simulink model "balance_car_with_NN"  (R2023b)
settings: Solver=VariableStepAuto  StartTime=0.0  StopTime=100  RelTol=1e-3
values from neighbouring files (symbols this model uses):
  d = 0.1612    [new_parameter.m]    (also in parameter.m)
  g = 9.8    [new_parameter.m]    (also in parameter.m)
  I = 0.5*m*r^2    (= 1.3475e-05)    [new_parameter.m]    (also in parameter.m = 1.97568e-05)
  J_delta = (1/12)*M*(0.0930^2+0.0530^2)    (= 0.000680796166667)    [new_parameter.m]    (also in parameter.m = 0.0006559705)
  J_p = (1/12)*M*(0.3^2+0.08^2)    (= 0.00572776666667)    [new_parameter.m]    (also in parameter.m = 0.0006276369025)
  l = 0.5*0.8    (= 0.4)    [new_parameter.m]    (also in parameter.m = 0.04515)
  M = 0.757-2*m    (= 0.713)    [new_parameter.m]    (also in parameter.m = 0.687)
  m = 0.022    [new_parameter.m]    (also in parameter.m = 0.035)
  r = 0.07/2    (= 0.035)    [new_parameter.m]    (also in parameter.m = 0.0336)
  T = evalin('base', 'T')    [NN_controller.m]    (also in new_parameter.m = 0.01; parameter.m = 0.02)
undefined symbols (not defined in the file or in its folder): now
libraries: slpidlib x7, simulink x6, cstblocks x1
settings Model: Creator=zhy  LastModifiedBy=zhy

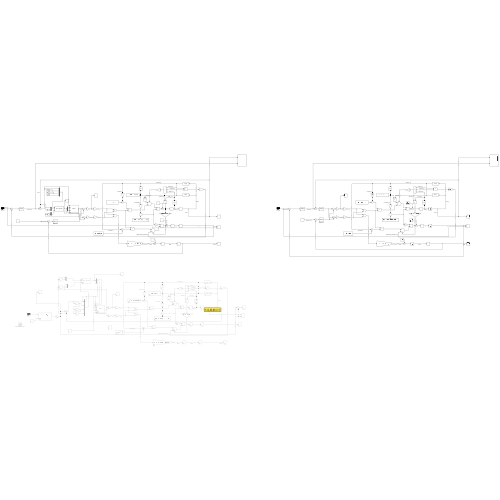
[thumbnail: Simulink's stored preview of the top-level diagram]
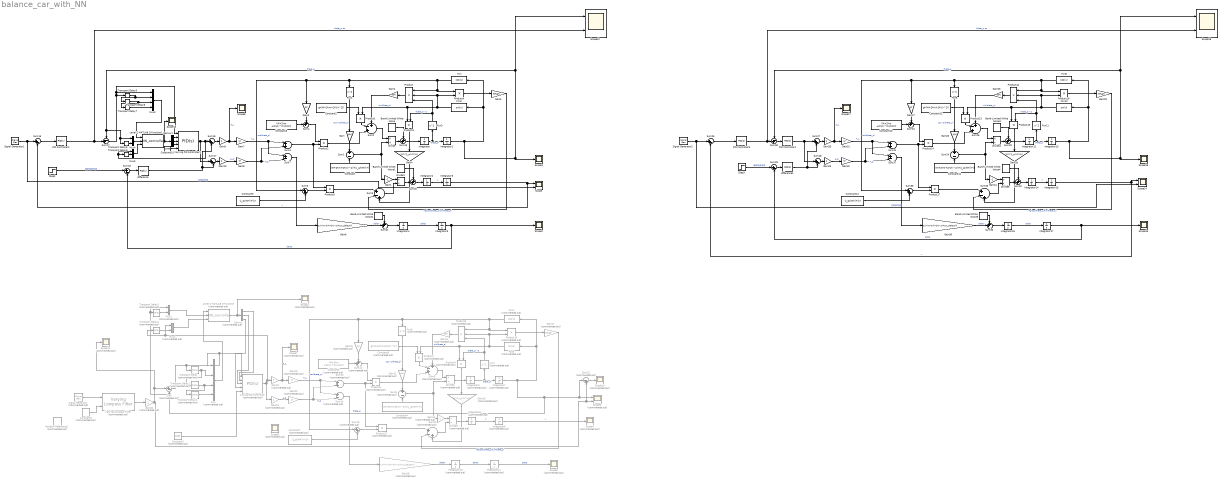
== system balance_car_with_NN ==
  Band-Limited White Noise : simulink/Sources/Band-Limited White Noise  Cov=[0.00001]  Ts=0.1  seed=[23341]
  Band-Limited White Noise1 : simulink/Sources/Band-Limited White Noise  Cov=[0.00001]  Ts=0.1  seed=[23342]
  Band-Limited White Noise2 : simulink/Sources/Band-Limited White Noise  Cov=[0.0001]  Ts=0.1  seed=[23343]
  Band-Limited White Noise3 : simulink/Sources/Band-Limited White Noise  Cov=[0.00001]  Ts=0.1  seed=[23341]
  Band-Limited White Noise4 : simulink/Sources/Band-Limited White Noise  Cov=[0.00001]  Ts=0.1  seed=[23342]
  Band-Limited White Noise5 : simulink/Sources/Band-Limited White Noise  Cov=[0.0001]  Ts=0.1  seed=[23343]
  Constant : Constant  Value=(M+2*m+2*I/(r^2))*(J_p/(M*l)+l)
  Constant1 : Constant  Commented=on  Value=1000
  Constant10 : Constant  Value=1000
  Constant11 : Constant  Value=(M+2*m+2*I/(r^2))*(J_p/(M*l)+l)
  Constant12 : Constant  Value=g*(M+2*m+2*I/(r^2))
  Constant13 : Constant  Value=(M+2*m +2*I/(r^2))/(M*l)
  Constant14 : Constant  Value=(J_p/(M*l)+l)/r
  Constant2 : Constant  Value=g*(M+2*m+2*I/(r^2))
  Constant3 : Constant  Value=(M+2*m +2*I/(r^2))/(M*l)
  Constant4 : Constant  Commented=on  Value=(M+2*m+2*I/(r^2))*(J_p/(M*l)+l)
  Constant5 : Constant  Commented=on  Value=g*(M+2*m+2*I/(r^2))
  Constant6 : Constant  Commented=on  Value=(M+2*m +2*I/(r^2))/(M*l)
  Constant7 : Constant  Commented=on  Value=(J_p/(M*l)+l)/r
  Constant8 : Constant  Commented=on  Value=0.05*pi
  Constant9 : Constant  Value=(J_p/(M*l)+l)/r
  Demux : Demux  Commented=on  Outputs=3
  Demux1 : Demux  Outputs=3
  Divide : Product  Inputs=*/
  Divide1 : Product  Inputs=/*
  Divide2 : Product  Commented=on  Inputs=*/
  Divide3 : Product  Commented=on  Inputs=/*
  Divide4 : Product  Inputs=*/
  Divide5 : Product  Inputs=/*
  Fcn : Fcn  Expr=cos(u)
  Fcn{1,3,9,11} (4 alike) : Fcn  Expr=u^2
  Fcn10 : Fcn  Expr=sin(u)
  Fcn2 : Fcn  Expr=sin(u)
  Fcn4 : Fcn  Commented=on  Expr=cos(u)
  Fcn5 : Fcn  Commented=on  Expr=u^2
  Fcn6 : Fcn  Commented=on  Expr=sin(u)
  Fcn7 : Fcn  Commented=on  Expr=u^2
  Fcn8 : Fcn  Expr=cos(u)
  Gain{,2,23,26} (4 alike) : Gain  Gain=M*l
  Gain1 : Gain  Gain=-1
  Gain{9..10,25,33} (4 alike) : Gain
  Gain11 : Gain  Commented=on  Gain=M*l
  Gain12 : Gain  Commented=on  Gain=-1
  Gain13 : Gain  Commented=on
  Gain14 : Gain  Commented=on  Gain=M*l
  Gain15 : Gain  Commented=on  Gain=1/r
  Gain16 : Gain  Commented=on  Gain=(M*l)*(J_p/(M*l)+l)
  Gain17 : Gain  Commented=on  Gain=M*g*l
  Gain18 : Gain  Commented=on  Gain=1/(r*(m*d+I*d/(r^2)+2*J_delta/d))
  Gain19 : Gain  Commented=on  Gain=I/r
  Gain20 : Gain  Commented=on  Gain=I/r
  Gain21 : Gain  Commented=on
  Gain22 : Gain  Commented=on
  Gain24 : Gain  Gain=-1
  Gain27 : Gain  Gain=1/r
  Gain28 : Gain  Gain=(M*l)*(J_p/(M*l)+l)
  Gain29 : Gain  Gain=M*g*l
  Gain3 : Gain  Gain=1/r
  Gain30 : Gain  Gain=1/(r*(m*d+I*d/(r^2)+2*J_delta/d))
  Gain{7..8,31..32} (4 alike) : Gain  Gain=I/r
  Gain4 : Gain  Gain=(M*l)*(J_p/(M*l)+l)
  Gain5 : Gain  Gain=M*g*l
  Gain6 : Gain  Gain=1/(r*(m*d+I*d/(r^2)+2*J_delta/d))
  Integrator{,1..5,12..17} (12 alike) : Integrator
  Integrator{6..11} (6 alike) : Integrator  Commented=on
  Level-2 MATLAB S-Function : M-S-Function  Commented=on  FunctionName=NN_controller
  Level-2 MATLAB S-Function1 : M-S-Function  FunctionName=NN_controller
  Mux : Mux  Commented=on
  Mux1 : Mux  Commented=on  Inputs=2
  Mux2 : Mux  Commented=on  Inputs=2
  Mux3 : Mux
  Mux4 : Mux  Inputs=2
  Mux5 : Mux  Inputs=2
  PID Controller1 : slpidlib/PID Controller  Controller=PID  Form=Parallel  TimeDomain=Continuous-time  UseExternalTs=off  SampleTime=-1  IntegratorMethod=Forward Euler  FilterMethod=Forward Euler  ControllerParametersSource=internal  P=-280  I=-200  UseKiTs=off  D=-120  N=100000  UseFilter=on  TunerSelectOption=Transfer Function Based (PID Tuner App)  InitialConditionSource=internal  InitialConditionForIntegrator=0  InitialConditionForFilter=0  DifferentiatorICPrevScaledInput=0  ExternalReset=none  TrackingMode=off  Kt=1  LimitOutput=off  SatLimitsSource=internal  UpperSaturationLimit=inf  LowerSaturationLimit=-inf  LinearizeAsGain=on  AntiWindupMode=none  Kb=1  LimitIntegrator=off  UpperIntegratorSaturationLimit=inf  LowerIntegratorSaturationLimit=-inf  POutMin=[]  POutMax=[]  IOutMin=[]  IOutMax=[]  DOutMin=[]  DOutMax=[]  NOutMin=[]  NOutMax=[]  SumOutMin=[]  SumOutMax=[]  SaturationOutMin=[]  SaturationOutMax=[]  PParamMin=[]  PParamMax=[]  IParamMin=[]  IParamMax=[]  DParamMin=[]  DParamMax=[]  NParamMin=[]  NParamMax=[]  KbParamMin=[]  KbParamMax=[]  KtParamMin=[]  KtParamMax=[]  KbOutMin=[]  KbOutMax=[]  KtOutMin=[]  KtOutMax=[]  IntegratorOutMin=[]  IntegratorOutMax=[]  FilterOutMin=[]  FilterOutMax=[]  SumI1OutMin=[]  SumI1OutMax=[]  SumI2OutMin=[]  SumI2OutMax=[]  SumI3OutMin=[]  SumI3OutMax=[]  SumI4OutMin=[]  SumI4OutMax=[]  SumDOutMin=[]  SumDOutMax=[]  DifferentiatorOutMin=[]  DifferentiatorOutMax=[]  FilterDiffOutCoefMin=[]  FilterDiffOutCoefMax=[]  ReciprocalOutMin=[]  ReciprocalOutMax=[]  SumDenOutMin=[]  SumDenOutMax=[]  SumNumOutMin=[]  SumNumOutMax=[]  DivideOutMin=[]  DivideOutMax=[]  UdiffTsProdOutMin=[]  UdiffTsProdOutMax=[]  NTsProdOutMin=[]  NTsProdOutMax=[]  UintegralTsProdOutMin=[]  UintegralTsProdOutMax=[]  UngainTsProdOutMin=[]  UngainTsProdOutMax=[]  ClampingZeroOutDataTypeStr=Inherit: Inherit via back propagation  ClampingZeroOutMin=[]  ClampingZeroOutMax=[]  FilterDenConstantOutDataTypeStr=Inherit: Inherit via back propagation  FilterDenConstantOutMin=[]  FilterDenConstantOutMax=[]  PCopyOutDataTypeStr=Inherit: Inherit via back propagation  PCopyOutMin=[]  PCopyOutMax=[]  NCopyOutDataTypeStr=Inherit: Inherit via back propagation  NCopyOutMin=[]  NCopyOutMax=[]  IntegratorContinuousStateAttributes=''  IntegratorStateMustResolveToSignalObject=off  IntegratorRTWStateStorageClass=Auto  FilterContinuousStateAttributes=''  FilterStateMustResolveToSignalObject=off  FilterRTWStateStorageClass=Auto  ParallelPVariant=InternalParameters  IdealPVariant=Disabled  IVariant=InternalParameters  DVariant=InternalParameters  IntegratorVariant=Continuous  SatVariant=Disabled  AWVariant=Passthrough  PCopyVariant=Disabled  TRVariant=Disabled  FdbkBlocksVariant=Forward  IdealPFdbkVariant=Disabled  SatFdbkVariant=Disabled  DerivativeFilterVariant=ContFilter  NVariant=InternalParameters  NCopyVariant=Disabled  FilterICVariant=InternalICsFilter  IntegratorICVariant=InternalICs  ExternalResetVariant=Disabled  TRSumVariant=Passthrough  SumFdbkVariant=Disabled  SumVariant=Sum_PID  TsampFilterVariant=InternalTs  TsampNgainVariant=Passthrough  TsampIntegralVariant=Disabled_SignalSpec  ExternalSaturationOutDataTypeStr=Inherit: Same as second input
  PID Controller2 : slpidlib/PID Controller  Controller=PID  Form=Parallel  TimeDomain=Continuous-time  UseExternalTs=off  SampleTime=-1  IntegratorMethod=Forward Euler  FilterMethod=Forward Euler  ControllerParametersSource=internal  P=0.01  I=0  UseKiTs=off  D=0.2  N=1  UseFilter=on  TunerSelectOption=Transfer Function Based (PID Tuner App)  InitialConditionSource=internal  InitialConditionForIntegrator=0  InitialConditionForFilter=0  DifferentiatorICPrevScaledInput=0  ExternalReset=none  TrackingMode=off  Kt=1  LimitOutput=off  SatLimitsSource=internal  UpperSaturationLimit=inf  LowerSaturationLimit=-inf  LinearizeAsGain=on  AntiWindupMode=none  Kb=1  LimitIntegrator=off  UpperIntegratorSaturationLimit=inf  LowerIntegratorSaturationLimit=-inf  POutMin=[]  POutMax=[]  IOutMin=[]  IOutMax=[]  DOutMin=[]  DOutMax=[]  NOutMin=[]  NOutMax=[]  SumOutMin=[]  SumOutMax=[]  SaturationOutMin=[]  SaturationOutMax=[]  PParamMin=[]  PParamMax=[]  IParamMin=[]  IParamMax=[]  DParamMin=[]  DParamMax=[]  NParamMin=[]  NParamMax=[]  KbParamMin=[]  KbParamMax=[]  KtParamMin=[]  KtParamMax=[]  KbOutMin=[]  KbOutMax=[]  KtOutMin=[]  KtOutMax=[]  IntegratorOutMin=[]  IntegratorOutMax=[]  FilterOutMin=[]  FilterOutMax=[]  SumI1OutMin=[]  SumI1OutMax=[]  SumI2OutMin=[]  SumI2OutMax=[]  SumI3OutMin=[]  SumI3OutMax=[]  SumI4OutMin=[]  SumI4OutMax=[]  SumDOutMin=[]  SumDOutMax=[]  DifferentiatorOutMin=[]  DifferentiatorOutMax=[]  FilterDiffOutCoefMin=[]  FilterDiffOutCoefMax=[]  ReciprocalOutMin=[]  ReciprocalOutMax=[]  SumDenOutMin=[]  SumDenOutMax=[]  SumNumOutMin=[]  SumNumOutMax=[]  DivideOutMin=[]  DivideOutMax=[]  UdiffTsProdOutMin=[]  UdiffTsProdOutMax=[]  NTsProdOutMin=[]  NTsProdOutMax=[]  UintegralTsProdOutMin=[]  UintegralTsProdOutMax=[]  UngainTsProdOutMin=[]  UngainTsProdOutMax=[]  ClampingZeroOutDataTypeStr=Inherit: Inherit via back propagation  ClampingZeroOutMin=[]  ClampingZeroOutMax=[]  FilterDenConstantOutDataTypeStr=Inherit: Inherit via back propagation  FilterDenConstantOutMin=[]  FilterDenConstantOutMax=[]  PCopyOutDataTypeStr=Inherit: Inherit via back propagation  PCopyOutMin=[]  PCopyOutMax=[]  NCopyOutDataTypeStr=Inherit: Inherit via back propagation  NCopyOutMin=[]  NCopyOutMax=[]  IntegratorContinuousStateAttributes=''  IntegratorStateMustResolveToSignalObject=off  IntegratorRTWStateStorageClass=Auto  FilterContinuousStateAttributes=''  FilterStateMustResolveToSignalObject=off  FilterRTWStateStorageClass=Auto  ParallelPVariant=InternalParameters  IdealPVariant=Disabled  IVariant=InternalParameters  DVariant=InternalParameters  IntegratorVariant=Continuous  SatVariant=Disabled  AWVariant=Passthrough  PCopyVariant=Disabled  TRVariant=Disabled  FdbkBlocksVariant=Forward  IdealPFdbkVariant=Disabled  SatFdbkVariant=Disabled  DerivativeFilterVariant=ContFilter  NVariant=InternalParameters  NCopyVariant=Disabled  FilterICVariant=InternalICsFilter  IntegratorICVariant=InternalICs  ExternalResetVariant=Disabled  TRSumVariant=Passthrough  SumFdbkVariant=Disabled  SumVariant=Sum_PID  TsampFilterVariant=InternalTs  TsampNgainVariant=Passthrough  TsampIntegralVariant=Disabled_SignalSpec  ExternalSaturationOutDataTypeStr=Inherit: Same as second input
  PID Controller3 : slpidlib/PID Controller  Controller=PID  Form=Parallel  TimeDomain=Continuous-time  UseExternalTs=off  SampleTime=-1  IntegratorMethod=Forward Euler  FilterMethod=Forward Euler  ControllerParametersSource=internal  P=0.01  I=0  UseKiTs=off  D=0.2  N=1  UseFilter=on  TunerSelectOption=Transfer Function Based (PID Tuner App)  InitialConditionSource=internal  InitialConditionForIntegrator=0  InitialConditionForFilter=0  DifferentiatorICPrevScaledInput=0  ExternalReset=none  TrackingMode=off  Kt=1  LimitOutput=off  SatLimitsSource=internal  UpperSaturationLimit=inf  LowerSaturationLimit=-inf  LinearizeAsGain=on  AntiWindupMode=none  Kb=1  LimitIntegrator=off  UpperIntegratorSaturationLimit=inf  LowerIntegratorSaturationLimit=-inf  POutMin=[]  POutMax=[]  IOutMin=[]  IOutMax=[]  DOutMin=[]  DOutMax=[]  NOutMin=[]  NOutMax=[]  SumOutMin=[]  SumOutMax=[]  SaturationOutMin=[]  SaturationOutMax=[]  PParamMin=[]  PParamMax=[]  IParamMin=[]  IParamMax=[]  DParamMin=[]  DParamMax=[]  NParamMin=[]  NParamMax=[]  KbParamMin=[]  KbParamMax=[]  KtParamMin=[]  KtParamMax=[]  KbOutMin=[]  KbOutMax=[]  KtOutMin=[]  KtOutMax=[]  IntegratorOutMin=[]  IntegratorOutMax=[]  FilterOutMin=[]  FilterOutMax=[]  SumI1OutMin=[]  SumI1OutMax=[]  SumI2OutMin=[]  SumI2OutMax=[]  SumI3OutMin=[]  SumI3OutMax=[]  SumI4OutMin=[]  SumI4OutMax=[]  SumDOutMin=[]  SumDOutMax=[]  DifferentiatorOutMin=[]  DifferentiatorOutMax=[]  FilterDiffOutCoefMin=[]  FilterDiffOutCoefMax=[]  ReciprocalOutMin=[]  ReciprocalOutMax=[]  SumDenOutMin=[]  SumDenOutMax=[]  SumNumOutMin=[]  SumNumOutMax=[]  DivideOutMin=[]  DivideOutMax=[]  UdiffTsProdOutMin=[]  UdiffTsProdOutMax=[]  NTsProdOutMin=[]  NTsProdOutMax=[]  UintegralTsProdOutMin=[]  UintegralTsProdOutMax=[]  UngainTsProdOutMin=[]  UngainTsProdOutMax=[]  ClampingZeroOutDataTypeStr=Inherit: Inherit via back propagation  ClampingZeroOutMin=[]  ClampingZeroOutMax=[]  FilterDenConstantOutDataTypeStr=Inherit: Inherit via back propagation  FilterDenConstantOutMin=[]  FilterDenConstantOutMax=[]  PCopyOutDataTypeStr=Inherit: Inherit via back propagation  PCopyOutMin=[]  PCopyOutMax=[]  NCopyOutDataTypeStr=Inherit: Inherit via back propagation  NCopyOutMin=[]  NCopyOutMax=[]  IntegratorContinuousStateAttributes=''  IntegratorStateMustResolveToSignalObject=off  IntegratorRTWStateStorageClass=Auto  FilterContinuousStateAttributes=''  FilterStateMustResolveToSignalObject=off  FilterRTWStateStorageClass=Auto  ParallelPVariant=InternalParameters  IdealPVariant=Disabled  IVariant=InternalParameters  DVariant=InternalParameters  IntegratorVariant=Continuous  SatVariant=Disabled  AWVariant=Passthrough  PCopyVariant=Disabled  TRVariant=Disabled  FdbkBlocksVariant=Forward  IdealPFdbkVariant=Disabled  SatFdbkVariant=Disabled  DerivativeFilterVariant=ContFilter  NVariant=InternalParameters  NCopyVariant=Disabled  FilterICVariant=InternalICsFilter  IntegratorICVariant=InternalICs  ExternalResetVariant=Disabled  TRSumVariant=Passthrough  SumFdbkVariant=Disabled  SumVariant=Sum_PID  TsampFilterVariant=InternalTs  TsampNgainVariant=Passthrough  TsampIntegralVariant=Disabled_SignalSpec  ExternalSaturationOutDataTypeStr=Inherit: Same as second input
  Product : Product  Inputs=3
  Product{1..5,13..17} (10 alike) : Product
  Product{7..11} (5 alike) : Product  Commented=on
  Product12 : Product  Inputs=3
  Product6 : Product  Commented=on  Inputs=3
  Random Reference2 : UniformRandomNumber  Commented=on  Minimum=-0.01  Maximum=0.01  Seed=round(now)  SampleTime=8
  Scope{,12,14,18} (4 alike) : Scope  NumInputPorts=2
  Scope{1,4..5,7,9..11} (7 alike) : Scope  Commented=on
  Scope{2..3,8,13,15..17} (7 alike) : Scope
  Scope6 : Scope  Commented=on  NumInputPorts=2
  Signal Generator : SignalGenerator  Commented=on  Amplitude=0.5  Frequency=0.01
  Signal Generator1 : SignalGenerator  Amplitude=0.2  Frequency=0.05
  Signal Generator2 : SignalGenerator  Amplitude=0.2  Frequency=0.05
  Step2 : Step  Time=20  After=0.1  SampleTime=0
  Step3 : Step  Time=20  After=0.1  SampleTime=0
  Sum : Sum  Commented=on  Inputs=|+-
  Sum1 : Sum  Inputs=+-
  Sum10 : Sum  Commented=on  Inputs=|++|
  Sum11 : Sum  Commented=on  Inputs=++|
  Sum12 : Sum  Commented=on  Inputs=|+-+
  Sum13 : Sum  Commented=on  Inputs=|++
  Sum14 : Sum  Commented=on  Inputs=|+-|
  Sum{15,17..18,26,28..29} (6 alike) : Sum  Inputs=|+-
  Sum{6,16,27,36} (4 alike) : Sum  Inputs=|++
  Sum{4,19..21,30,32..34} (8 alike) : Sum  Inputs=++|
  Sum2 : Sum  Inputs=+-+|
  Sum22 : Sum  Commented=on  Inputs=|-+
  Sum23 : Sum  Inputs=-+|
  Sum24 : Sum  Inputs=+-
  Sum25 : Sum  Inputs=+-+|
  Sum3 : Sum  Inputs=|++|
  Sum31 : Sum  Inputs=|++|
  Sum35 : Sum  Inputs=|+-+
  Sum37 : Sum  Inputs=|+-|
  Sum38 : Sum  Inputs=-+|
  Sum5 : Sum  Inputs=|+-+
  Sum7 : Sum  Inputs=|+-|
  Sum8 : Sum  Commented=on  Inputs=+-
  Sum9 : Sum  Commented=on  Inputs=+-+|
  Transport Delay{,1..4} (5 alike) : TransportDelay  Commented=on  DelayTime=T  BufferSize=8192
  Transport Delay{5..9} (5 alike) : TransportDelay  DelayTime=T  BufferSize=8192
  Varying Lowpass Filter : cstblocks/Linear Parameter Varying/Varying Lowpass Filter  Commented=on  N=2
  Varying PID Controller : slpidlib/PID Controller  Commented=on  Controller=PID  Form=Parallel  TimeDomain=Continuous-time  UseExternalTs=off  SampleTime=-1  IntegratorMethod=Forward Euler  FilterMethod=Forward Euler  ControllerParametersSource=external  P=1  I=1  UseKiTs=off  D=0  N=100  UseFilter=on  TunerSelectOption=Transfer Function Based (PID Tuner App)  InitialConditionSource=internal  InitialConditionForIntegrator=0  InitialConditionForFilter=0  DifferentiatorICPrevScaledInput=0  ExternalReset=none  TrackingMode=off  Kt=1  LimitOutput=off  SatLimitsSource=internal  UpperSaturationLimit=inf  LowerSaturationLimit=-inf  LinearizeAsGain=on  AntiWindupMode=none  Kb=1  LimitIntegrator=off  UpperIntegratorSaturationLimit=inf  LowerIntegratorSaturationLimit=-inf  POutMin=[]  POutMax=[]  IOutMin=[]  IOutMax=[]  DOutMin=[]  DOutMax=[]  NOutMin=[]  NOutMax=[]  SumOutMin=[]  SumOutMax=[]  SaturationOutMin=[]  SaturationOutMax=[]  PParamMin=[]  PParamMax=[]  IParamMin=[]  IParamMax=[]  DParamMin=[]  DParamMax=[]  NParamMin=[]  NParamMax=[]  KbParamMin=[]  KbParamMax=[]  KtParamMin=[]  KtParamMax=[]  KbOutMin=[]  KbOutMax=[]  KtOutMin=[]  KtOutMax=[]  IntegratorOutMin=[]  IntegratorOutMax=[]  FilterOutMin=[]  FilterOutMax=[]  SumI1OutMin=[]  SumI1OutMax=[]  SumI2OutMin=[]  SumI2OutMax=[]  SumI3OutMin=[]  SumI3OutMax=[]  SumI4OutMin=[]  SumI4OutMax=[]  SumDOutMin=[]  SumDOutMax=[]  DifferentiatorOutMin=[]  DifferentiatorOutMax=[]  FilterDiffOutCoefMin=[]  FilterDiffOutCoefMax=[]  ReciprocalOutMin=[]  ReciprocalOutMax=[]  SumDenOutMin=[]  SumDenOutMax=[]  SumNumOutMin=[]  SumNumOutMax=[]  DivideOutMin=[]  DivideOutMax=[]  UdiffTsProdOutMin=[]  UdiffTsProdOutMax=[]  NTsProdOutMin=[]  NTsProdOutMax=[]  UintegralTsProdOutMin=[]  UintegralTsProdOutMax=[]  UngainTsProdOutMin=[]  UngainTsProdOutMax=[]  ClampingZeroOutDataTypeStr=Inherit: Inherit via back propagation  ClampingZeroOutMin=[]  ClampingZeroOutMax=[]  FilterDenConstantOutDataTypeStr=Inherit: Inherit via back propagation  FilterDenConstantOutMin=[]  FilterDenConstantOutMax=[]  PCopyOutDataTypeStr=Inherit: Inherit via back propagation  PCopyOutMin=[]  PCopyOutMax=[]  NCopyOutDataTypeStr=Inherit: Inherit via back propagation  NCopyOutMin=[]  NCopyOutMax=[]  IntegratorContinuousStateAttributes=''  IntegratorStateMustResolveToSignalObject=off  IntegratorRTWStateStorageClass=Auto  FilterContinuousStateAttributes=''  FilterStateMustResolveToSignalObject=off  FilterRTWStateStorageClass=Auto  ParallelPVariant=ExternalParameters  IdealPVariant=Disabled  IVariant=ExternalParameters  DVariant=ExternalParameters  IntegratorVariant=Continuous  SatVariant=Disabled  AWVariant=Passthrough  PCopyVariant=Disabled  TRVariant=Disabled  FdbkBlocksVariant=Forward  IdealPFdbkVariant=Disabled  SatFdbkVariant=Disabled  DerivativeFilterVariant=ContFilter  NVariant=ExternalParameters  NCopyVariant=Disabled  FilterICVariant=InternalICsFilter  IntegratorICVariant=InternalICs  ExternalResetVariant=Disabled  TRSumVariant=Passthrough  SumFdbkVariant=Disabled  SumVariant=Sum_PID  TsampFilterVariant=InternalTs  TsampNgainVariant=Passthrough  TsampIntegralVariant=Disabled_SignalSpec  ExternalSaturationOutDataTypeStr=Inherit: Same as second input
      settings: LibrarySourceBlock=cstblocks/Linear Parameter Varying/Varying PID Controller
  Varying PID Controller1 : slpidlib/PID Controller  Controller=PID  Form=Parallel  TimeDomain=Continuous-time  UseExternalTs=off  SampleTime=-1  IntegratorMethod=Forward Euler  FilterMethod=Forward Euler  ControllerParametersSource=external  P=1  I=1  UseKiTs=off  D=0  N=100  UseFilter=on  TunerSelectOption=Transfer Function Based (PID Tuner App)  InitialConditionSource=internal  InitialConditionForIntegrator=0  InitialConditionForFilter=0  DifferentiatorICPrevScaledInput=0  ExternalReset=none  TrackingMode=off  Kt=1  LimitOutput=off  SatLimitsSource=internal  UpperSaturationLimit=inf  LowerSaturationLimit=-inf  LinearizeAsGain=on  AntiWindupMode=none  Kb=1  LimitIntegrator=off  UpperIntegratorSaturationLimit=inf  LowerIntegratorSaturationLimit=-inf  POutMin=[]  POutMax=[]  IOutMin=[]  IOutMax=[]  DOutMin=[]  DOutMax=[]  NOutMin=[]  NOutMax=[]  SumOutMin=[]  SumOutMax=[]  SaturationOutMin=[]  SaturationOutMax=[]  PParamMin=[]  PParamMax=[]  IParamMin=[]  IParamMax=[]  DParamMin=[]  DParamMax=[]  NParamMin=[]  NParamMax=[]  KbParamMin=[]  KbParamMax=[]  KtParamMin=[]  KtParamMax=[]  KbOutMin=[]  KbOutMax=[]  KtOutMin=[]  KtOutMax=[]  IntegratorOutMin=[]  IntegratorOutMax=[]  FilterOutMin=[]  FilterOutMax=[]  SumI1OutMin=[]  SumI1OutMax=[]  SumI2OutMin=[]  SumI2OutMax=[]  SumI3OutMin=[]  SumI3OutMax=[]  SumI4OutMin=[]  SumI4OutMax=[]  SumDOutMin=[]  SumDOutMax=[]  DifferentiatorOutMin=[]  DifferentiatorOutMax=[]  FilterDiffOutCoefMin=[]  FilterDiffOutCoefMax=[]  ReciprocalOutMin=[]  ReciprocalOutMax=[]  SumDenOutMin=[]  SumDenOutMax=[]  SumNumOutMin=[]  SumNumOutMax=[]  DivideOutMin=[]  DivideOutMax=[]  UdiffTsProdOutMin=[]  UdiffTsProdOutMax=[]  NTsProdOutMin=[]  NTsProdOutMax=[]  UintegralTsProdOutMin=[]  UintegralTsProdOutMax=[]  UngainTsProdOutMin=[]  UngainTsProdOutMax=[]  ClampingZeroOutDataTypeStr=Inherit: Inherit via back propagation  ClampingZeroOutMin=[]  ClampingZeroOutMax=[]  FilterDenConstantOutDataTypeStr=Inherit: Inherit via back propagation  FilterDenConstantOutMin=[]  FilterDenConstantOutMax=[]  PCopyOutDataTypeStr=Inherit: Inherit via back propagation  PCopyOutMin=[]  PCopyOutMax=[]  NCopyOutDataTypeStr=Inherit: Inherit via back propagation  NCopyOutMin=[]  NCopyOutMax=[]  IntegratorContinuousStateAttributes=''  IntegratorStateMustResolveToSignalObject=off  IntegratorRTWStateStorageClass=Auto  FilterContinuousStateAttributes=''  FilterStateMustResolveToSignalObject=off  FilterRTWStateStorageClass=Auto  ParallelPVariant=ExternalParameters  IdealPVariant=Disabled  IVariant=ExternalParameters  DVariant=ExternalParameters  IntegratorVariant=Continuous  SatVariant=Disabled  AWVariant=Passthrough  PCopyVariant=Disabled  TRVariant=Disabled  FdbkBlocksVariant=Forward  IdealPFdbkVariant=Disabled  SatFdbkVariant=Disabled  DerivativeFilterVariant=ContFilter  NVariant=ExternalParameters  NCopyVariant=Disabled  FilterICVariant=InternalICsFilter  IntegratorICVariant=InternalICs  ExternalResetVariant=Disabled  TRSumVariant=Passthrough  SumFdbkVariant=Disabled  SumVariant=Sum_PID  TsampFilterVariant=InternalTs  TsampNgainVariant=Passthrough  TsampIntegralVariant=Disabled_SignalSpec  ExternalSaturationOutDataTypeStr=Inherit: Same as second input
      settings: LibrarySourceBlock=cstblocks/Linear Parameter Varying/Varying PID Controller
  difference : slpidlib/PID Controller  Controller=PID  Form=Parallel  TimeDomain=Continuous-time  UseExternalTs=off  SampleTime=-1  IntegratorMethod=Forward Euler  FilterMethod=Forward Euler  ControllerParametersSource=internal  P=1  I=0  UseKiTs=off  D=0.8  N=100000  UseFilter=on  TunerSelectOption=Transfer Function Based (PID Tuner App)  InitialConditionSource=internal  InitialConditionForIntegrator=0  InitialConditionForFilter=0  DifferentiatorICPrevScaledInput=0  ExternalReset=none  TrackingMode=off  Kt=1  LimitOutput=off  SatLimitsSource=internal  UpperSaturationLimit=inf  LowerSaturationLimit=-inf  LinearizeAsGain=on  AntiWindupMode=none  Kb=1  LimitIntegrator=off  UpperIntegratorSaturationLimit=inf  LowerIntegratorSaturationLimit=-inf  POutMin=[]  POutMax=[]  IOutMin=[]  IOutMax=[]  DOutMin=[]  DOutMax=[]  NOutMin=[]  NOutMax=[]  SumOutMin=[]  SumOutMax=[]  SaturationOutMin=[]  SaturationOutMax=[]  PParamMin=[]  PParamMax=[]  IParamMin=[]  IParamMax=[]  DParamMin=[]  DParamMax=[]  NParamMin=[]  NParamMax=[]  KbParamMin=[]  KbParamMax=[]  KtParamMin=[]  KtParamMax=[]  KbOutMin=[]  KbOutMax=[]  KtOutMin=[]  KtOutMax=[]  IntegratorOutMin=[]  IntegratorOutMax=[]  FilterOutMin=[]  FilterOutMax=[]  SumI1OutMin=[]  SumI1OutMax=[]  SumI2OutMin=[]  SumI2OutMax=[]  SumI3OutMin=[]  SumI3OutMax=[]  SumI4OutMin=[]  SumI4OutMax=[]  SumDOutMin=[]  SumDOutMax=[]  DifferentiatorOutMin=[]  DifferentiatorOutMax=[]  FilterDiffOutCoefMin=[]  FilterDiffOutCoefMax=[]  ReciprocalOutMin=[]  ReciprocalOutMax=[]  SumDenOutMin=[]  SumDenOutMax=[]  SumNumOutMin=[]  SumNumOutMax=[]  DivideOutMin=[]  DivideOutMax=[]  UdiffTsProdOutMin=[]  UdiffTsProdOutMax=[]  NTsProdOutMin=[]  NTsProdOutMax=[]  UintegralTsProdOutMin=[]  UintegralTsProdOutMax=[]  UngainTsProdOutMin=[]  UngainTsProdOutMax=[]  ClampingZeroOutDataTypeStr=Inherit: Inherit via back propagation  ClampingZeroOutMin=[]  ClampingZeroOutMax=[]  FilterDenConstantOutDataTypeStr=Inherit: Inherit via back propagation  FilterDenConstantOutMin=[]  FilterDenConstantOutMax=[]  PCopyOutDataTypeStr=Inherit: Inherit via back propagation  PCopyOutMin=[]  PCopyOutMax=[]  NCopyOutDataTypeStr=Inherit: Inherit via back propagation  NCopyOutMin=[]  NCopyOutMax=[]  IntegratorContinuousStateAttributes=''  IntegratorStateMustResolveToSignalObject=off  IntegratorRTWStateStorageClass=Auto  FilterContinuousStateAttributes=''  FilterStateMustResolveToSignalObject=off  FilterRTWStateStorageClass=Auto  ParallelPVariant=InternalParameters  IdealPVariant=Disabled  IVariant=InternalParameters  DVariant=InternalParameters  IntegratorVariant=Continuous  SatVariant=Disabled  AWVariant=Passthrough  PCopyVariant=Disabled  TRVariant=Disabled  FdbkBlocksVariant=Forward  IdealPFdbkVariant=Disabled  SatFdbkVariant=Disabled  DerivativeFilterVariant=ContFilter  NVariant=InternalParameters  NCopyVariant=Disabled  FilterICVariant=InternalICsFilter  IntegratorICVariant=InternalICs  ExternalResetVariant=Disabled  TRSumVariant=Passthrough  SumFdbkVariant=Disabled  SumVariant=Sum_PID  TsampFilterVariant=InternalTs  TsampNgainVariant=Passthrough  TsampIntegralVariant=Disabled_SignalSpec  ExternalSaturationOutDataTypeStr=Inherit: Same as second input
  difference1 : slpidlib/PID Controller  Controller=PID  Form=Parallel  TimeDomain=Continuous-time  UseExternalTs=off  SampleTime=-1  IntegratorMethod=Forward Euler  FilterMethod=Forward Euler  ControllerParametersSource=internal  P=1  I=0  UseKiTs=off  D=0.8  N=100000  UseFilter=on  TunerSelectOption=Transfer Function Based (PID Tuner App)  InitialConditionSource=internal  InitialConditionForIntegrator=0  InitialConditionForFilter=0  DifferentiatorICPrevScaledInput=0  ExternalReset=none  TrackingMode=off  Kt=1  LimitOutput=off  SatLimitsSource=internal  UpperSaturationLimit=inf  LowerSaturationLimit=-inf  LinearizeAsGain=on  AntiWindupMode=none  Kb=1  LimitIntegrator=off  UpperIntegratorSaturationLimit=inf  LowerIntegratorSaturationLimit=-inf  POutMin=[]  POutMax=[]  IOutMin=[]  IOutMax=[]  DOutMin=[]  DOutMax=[]  NOutMin=[]  NOutMax=[]  SumOutMin=[]  SumOutMax=[]  SaturationOutMin=[]  SaturationOutMax=[]  PParamMin=[]  PParamMax=[]  IParamMin=[]  IParamMax=[]  DParamMin=[]  DParamMax=[]  NParamMin=[]  NParamMax=[]  KbParamMin=[]  KbParamMax=[]  KtParamMin=[]  KtParamMax=[]  KbOutMin=[]  KbOutMax=[]  KtOutMin=[]  KtOutMax=[]  IntegratorOutMin=[]  IntegratorOutMax=[]  FilterOutMin=[]  FilterOutMax=[]  SumI1OutMin=[]  SumI1OutMax=[]  SumI2OutMin=[]  SumI2OutMax=[]  SumI3OutMin=[]  SumI3OutMax=[]  SumI4OutMin=[]  SumI4OutMax=[]  SumDOutMin=[]  SumDOutMax=[]  DifferentiatorOutMin=[]  DifferentiatorOutMax=[]  FilterDiffOutCoefMin=[]  FilterDiffOutCoefMax=[]  ReciprocalOutMin=[]  ReciprocalOutMax=[]  SumDenOutMin=[]  SumDenOutMax=[]  SumNumOutMin=[]  SumNumOutMax=[]  DivideOutMin=[]  DivideOutMax=[]  UdiffTsProdOutMin=[]  UdiffTsProdOutMax=[]  NTsProdOutMin=[]  NTsProdOutMax=[]  UintegralTsProdOutMin=[]  UintegralTsProdOutMax=[]  UngainTsProdOutMin=[]  UngainTsProdOutMax=[]  ClampingZeroOutDataTypeStr=Inherit: Inherit via back propagation  ClampingZeroOutMin=[]  ClampingZeroOutMax=[]  FilterDenConstantOutDataTypeStr=Inherit: Inherit via back propagation  FilterDenConstantOutMin=[]  FilterDenConstantOutMax=[]  PCopyOutDataTypeStr=Inherit: Inherit via back propagation  PCopyOutMin=[]  PCopyOutMax=[]  NCopyOutDataTypeStr=Inherit: Inherit via back propagation  NCopyOutMin=[]  NCopyOutMax=[]  IntegratorContinuousStateAttributes=''  IntegratorStateMustResolveToSignalObject=off  IntegratorRTWStateStorageClass=Auto  FilterContinuousStateAttributes=''  FilterStateMustResolveToSignalObject=off  FilterRTWStateStorageClass=Auto  ParallelPVariant=InternalParameters  IdealPVariant=Disabled  IVariant=InternalParameters  DVariant=InternalParameters  IntegratorVariant=Continuous  SatVariant=Disabled  AWVariant=Passthrough  PCopyVariant=Disabled  TRVariant=Disabled  FdbkBlocksVariant=Forward  IdealPFdbkVariant=Disabled  SatFdbkVariant=Disabled  DerivativeFilterVariant=ContFilter  NVariant=InternalParameters  NCopyVariant=Disabled  FilterICVariant=InternalICsFilter  IntegratorICVariant=InternalICs  ExternalResetVariant=Disabled  TRSumVariant=Passthrough  SumFdbkVariant=Disabled  SumVariant=Sum_PID  TsampFilterVariant=InternalTs  TsampNgainVariant=Passthrough  TsampIntegralVariant=Disabled_SignalSpec  ExternalSaturationOutDataTypeStr=Inherit: Same as second input
  wires:
  Constant8/1 -> Varying Lowpass Filter/2
  Gain22/1 -> Sum22/2, Scope6/2, Scope11/1, Sum/1
  Varying Lowpass Filter/1 -> Gain22/1
  Signal Generator/1 -> Varying Lowpass Filter/1
  Gain15/1 -> Sum11/1
  Product8/1 -> Sum9/3
  Product7/1 -> Sum9/2
  Sum22/1 -> Scope10/1
  Divide2/1 -> Integrator6/1
  Constant7/1 -> Sum13/2
  Gain19/1 -> Sum14/1, Sum10/1  "T_L"
  Sum8/1 -> Gain12/1, Divide2/2
  Fcn7/1 -> Product6/3, Product9/2  "theta_p'^2"
  Integrator9/1 -> Scope4/1  "x"
  Integrator8/1 -> Integrator9/1  "x'"
  Gain12/1 -> Divide3/1
  Product10/1 -> Gain17/1
  Gain17/1 -> Sum12/2  "Mglcos(theta_p)sin(theta_p)"
  Fcn4/1 -> Product10/1, Product6/1, Fcn5/1, Sum13/1, Gain15/1  "cos(theta_p)"
  Gain14/1 -> Sum9/1
  Gain11/1 -> Sum8/1
  Divide3/1 -> Integrator8/1
  Sum11/1 -> Product8/1
  Product11/1 -> Sum12/1
  Product9/1 -> Gain16/1
  Gain18/1 -> Integrator10/1  "delta''"
  Sum13/1 -> Product11/2
  Sum10/1 -> Product11/1, Product8/2
  Constant4/1 -> Sum8/2
  Constant5/1 -> Product7/1
  Sum12/1 -> Divide3/2
  Integrator6/1 -> Integrator7/1, Fcn7/1  "theta_p'"
  Fcn5/1 -> Gain11/1  "cos^2(theta_p)"
  Integrator10/1 -> Integrator11/1  "delta'"
  Gain13/1 -> Gain20/1  "a_R"
  Integrator11/1 -> Scope5/1  "delta"
  Gain20/1 -> Sum14/2, Sum10/2  "T_R"
  Integrator7/1 -> Transport Delay3/1, Mux1/1, Sum/2, Sum22/1, Scope6/1, Fcn6/1, Fcn4/1  "theta_p"
  Gain21/1 -> Scope7/1, Gain19/1  "a_L"
  Fcn6/1 -> Product7/2, Product9/1, Product10/2, Product6/2  "sin(theta_p)"
  Constant6/1 -> Sum11/2
  Sum9/1 -> Divide2/1
  Sum14/1 -> Gain18/1
  Product6/1 -> Gain14/1
  Gain16/1 -> Sum12/3
  Mux/1 -> Level-2 MATLAB S-Function/1
  Sum/1 -> Varying PID Controller/1, Mux/1, Transport Delay/1
  Transport Delay/1 -> Mux/2, Transport Delay1/1
  Transport Delay1/1 -> Transport Delay2/1, Mux/3
  Transport Delay2/1 -> Mux/4
  Level-2 MATLAB S-Function/1 -> Scope1/1, Demux/1
  Varying PID Controller/1 -> Transport Delay4/1, Mux2/1, Gain21/1, Gain13/1
  Demux/1 -> Varying PID Controller/2
  Demux/2 -> Varying PID Controller/3
  Demux/3 -> Varying PID Controller/4
  Constant1/1 -> Varying PID Controller/5
  Mux1/1 -> Level-2 MATLAB S-Function/2
  Mux2/1 -> Level-2 MATLAB S-Function/3
  Transport Delay3/1 -> Mux1/2
  Transport Delay4/1 -> Mux2/2
  Band-Limited White Noise2/1 -> Sum21/1
  Gain5/1 -> Sum5/2  "Mglcos(theta_p)sin(theta_p)"
  Gain6/1 -> Sum21/2  "delta''"
  Sum6/1 -> Product5/2
  Integrator/1 -> Integrator1/1, Fcn3/1  "theta_p'"
  Sum21/1 -> Integrator4/1
  Band-Limited White Noise1/1 -> Sum20/1
  Product2/1 -> Sum2/3
  Sum20/1 -> Integrator2/1
  Divide/1 -> Sum19/2
  Step2/1 -> Sum18/1  "偏航角参考值"
  Divide1/1 -> Sum20/2
  difference/1 -> Sum16/2, Sum17/2
  Sum19/1 -> Integrator/1
  Band-Limited White Noise/1 -> Sum19/1
  Sum16/1 -> Gain9/1
  Sum15/1 -> PID Controller2/1
  Product4/1 -> Gain5/1
  Sum17/1 -> Gain10/1
  Integrator3/1 -> Sum15/2, Scope/1  "x"
  Gain3/1 -> Sum4/1
  PID Controller2/1 -> Scope12/2, Sum23/2  "theta_p sp"
  Fcn2/1 -> Product1/2, Product3/1, Product4/2, Product/2  "sin(theta_p)"
  Signal Generator1/1 -> Scope/2, Sum15/1  "位移参考值"
  Product1/1 -> Sum2/2
  Gain10/1 -> Gain8/1  "a_R"
  Product5/1 -> Sum5/1
  Gain4/1 -> Sum5/3
  Sum7/1 -> Gain6/1
  Sum1/1 -> Gain1/1, Divide/2
  Gain8/1 -> Sum7/2, Sum3/2  "T_R"
  Sum5/1 -> Divide1/2
  Gain7/1 -> Sum7/1, Sum3/1  "T_L"
  Varying PID Controller1/1 -> Transport Delay9/1, Mux5/1, Sum16/1, Sum17/1
  Constant3/1 -> Sum4/2
  Gain9/1 -> Scope8/1, Gain7/1  "a_L"
  Sum2/1 -> Divide/1
  Gain2/1 -> Sum2/1
  Fcn3/1 -> Product/3, Product3/2  "theta_p'^2"
  Constant/1 -> Sum1/2
  Gain1/1 -> Divide1/1
  Product/1 -> Gain2/1
  Sum3/1 -> Product5/1, Product2/2
  Constant9/1 -> Sum6/2
  Integrator4/1 -> Integrator5/1  "delta'"
  Product3/1 -> Gain4/1
  Fcn1/1 -> Gain/1  "cos^2(theta_p)"
  Integrator1/1 -> Scope12/1, Mux4/1, Transport Delay8/1, Sum23/1, Scope3/1, Fcn2/1, Fcn/1  "theta_p"
  Integrator2/1 -> Integrator3/1  "x'"
  Sum4/1 -> Product2/1
  Constant2/1 -> Product1/1
  Gain/1 -> Sum1/1
  Fcn/1 -> Product4/1, Product/1, Fcn1/1, Sum6/1, Gain3/1  "cos(theta_p)"
  Integrator5/1 -> Scope2/1, Sum18/2  "delta"
  Level-2 MATLAB S-Function1/1 -> Demux1/1, Scope13/1
  Demux1/1 -> Varying PID Controller1/2
  Demux1/2 -> Varying PID Controller1/3
  Demux1/3 -> Varying PID Controller1/4
  Constant10/1 -> Varying PID Controller1/5
  Transport Delay7/1 -> Mux3/4
  Transport Delay6/1 -> Transport Delay7/1, Mux3/3
  Transport Delay5/1 -> Transport Delay6/1, Mux3/2
  Sum23/1 -> Varying PID Controller1/1, Mux3/1, Transport Delay5/1
  Mux3/1 -> Level-2 MATLAB S-Function1/1
  Transport Delay8/1 -> Mux4/2
  Mux4/1 -> Level-2 MATLAB S-Function1/2
  Transport Delay9/1 -> Mux5/2
  Mux5/1 -> Level-2 MATLAB S-Function1/3
  Sum18/1 -> difference/1
  Band-Limited White Noise5/1 -> Sum33/1
  Gain29/1 -> Sum35/2  "Mglcos(theta_p)sin(theta_p)"
  Gain30/1 -> Sum33/2  "delta''"
  Sum36/1 -> Product17/2
  Integrator12/1 -> Integrator13/1, Fcn11/1  "theta_p'"
  Sum33/1 -> Integrator16/1
  Band-Limited White Noise4/1 -> Sum32/1
  Product14/1 -> Sum25/3
  Sum32/1 -> Integrator14/1
  Divide4/1 -> Sum30/2
  Step3/1 -> Sum29/1  "偏航角参考值"
  Sum38/1 -> PID Controller1/1
  Divide5/1 -> Sum32/2
  difference1/1 -> Sum27/2, Sum28/2
  Sum30/1 -> Integrator12/1
  Band-Limited White Noise3/1 -> Sum30/1
  Sum27/1 -> Gain33/1
  Sum26/1 -> PID Controller3/1
  Product16/1 -> Gain29/1
  Sum28/1 -> Gain25/1
  Integrator15/1 -> Scope14/1, Sum26/2  "x"
  Gain27/1 -> Sum34/1
  PID Controller3/1 -> Scope18/2, Sum38/2  "theta_p sp"
  Fcn10/1 -> Product13/2, Product15/1, Product16/2, Product12/2  "sin(theta_p)"
  Signal Generator2/1 -> Scope14/2, Sum26/1  "位移参考值"
  Product13/1 -> Sum25/2
  Gain25/1 -> Gain32/1  "a_R"
  Product17/1 -> Sum35/1
  Gain28/1 -> Sum35/3
  Sum29/1 -> difference1/1
  Sum37/1 -> Gain30/1
  Sum24/1 -> Gain24/1, Divide4/2
  Gain32/1 -> Sum37/2, Sum31/2  "T_R"
  Sum35/1 -> Divide5/2
  Gain31/1 -> Sum37/1, Sum31/1  "T_L"
  PID Controller1/1 -> Sum27/1, Sum28/1
  Constant13/1 -> Sum34/2
  Gain33/1 -> Scope17/1, Gain31/1  "a_L"
  Sum25/1 -> Divide4/1
  Gain26/1 -> Sum25/1
  Fcn11/1 -> Product12/3, Product15/2  "theta_p'^2"
  Constant11/1 -> Sum24/2
  Gain24/1 -> Divide5/1
  Product12/1 -> Gain26/1
  Sum31/1 -> Product17/1, Product14/2
  Constant14/1 -> Sum36/2
  Integrator16/1 -> Integrator17/1  "delta'"
  Product15/1 -> Gain28/1
  Fcn9/1 -> Gain23/1  "cos^2(theta_p)"
  Integrator13/1 -> Scope18/1, Sum38/1, Scope16/1, Fcn10/1, Fcn8/1  "theta_p"
  Integrator14/1 -> Integrator15/1  "x'"
  Sum34/1 -> Product14/1
  Constant12/1 -> Product13/1
  Gain23/1 -> Sum24/1
  Fcn8/1 -> Product16/1, Product12/1, Fcn9/1, Sum36/1, Gain27/1  "cos(theta_p)"
  Integrator17/1 -> Scope15/1, Sum29/2  "delta"
